simulink model "driveguard_simulation"  (R2023a)
settings: Solver=ode4  StartTime=0.0  StopTime=60  FixedStep=0.1  RelTol=1e-3
libraries: SignalEditorBlockLib x3, simulink x2
settings Model: Creator=Pulkit  LastModifiedBy=Pulkit

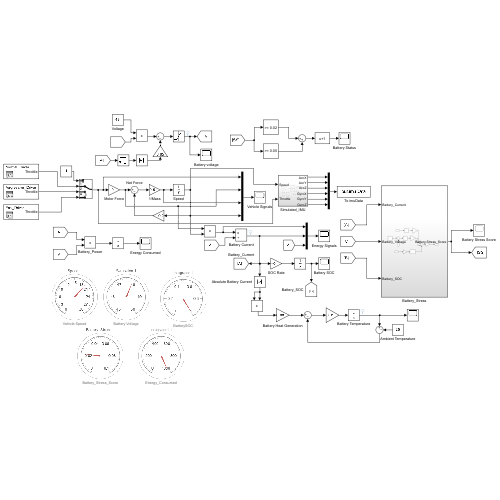
[thumbnail: Simulink's stored preview of the top-level diagram]
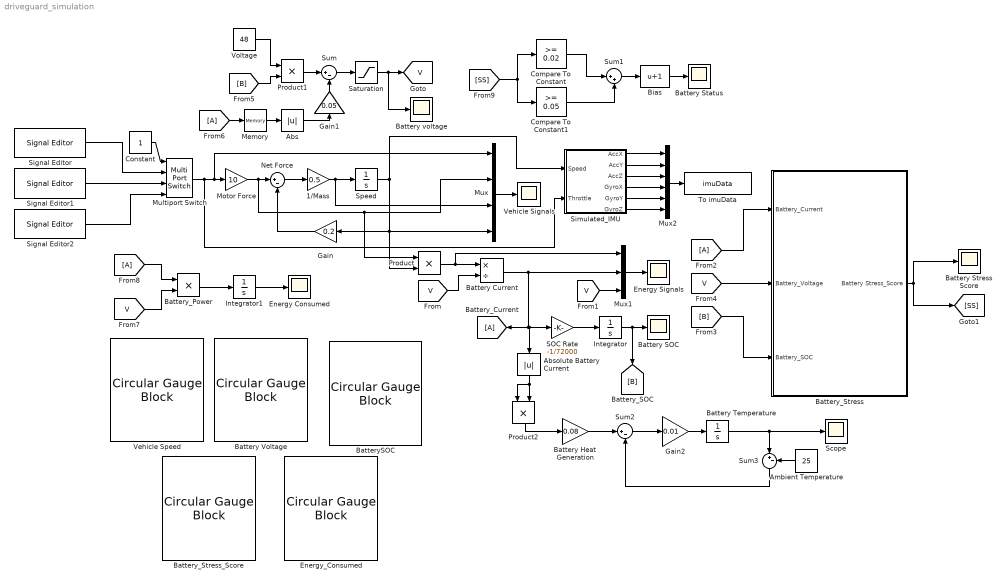
== system driveguard_simulation ==
  1/Mass : Gain  Gain=0.5
  Abs : Abs  SaturateOnIntegerOverflow=off
  Absolute Battery Current : Abs  SaturateOnIntegerOverflow=off
  Ambient Temperature : Constant  Value=25
  Battery Current : Product  Inputs=*/
  Battery Heat Generation : Gain  Gain=0.08
  Battery SOC : Scope
  Battery Status : Scope
  Battery Stress Score : Scope
  Battery Temperature : Integrator  InitialCondition=25
  Battery Voltage : CircularGaugeBlock  ScaleMin=45  ScaleMax=50  TickInterval=1
  Battery voltage : Scope
  BatterySOC : CircularGaugeBlock  ScaleMax=1  TickInterval=0.2
  Battery_Current : Goto
  Battery_Power : Product
  Battery_Stress : Subsystem
  Battery_Stress_Score : CircularGaugeBlock  ScaleMax=0.1  TickInterval=0.02
  Bias : Bias  Bias=1  SaturateOnIntegerOverflow=off
  Compare To Constant : simulink/Logic and Bit Operations/Compare To Constant  relop=>=  const=0.02  OutDataTypeStr=boolean
  Compare To Constant1 : simulink/Logic and Bit Operations/Compare To Constant  relop=>=  const=0.05  OutDataTypeStr=boolean
  Constant : Constant  SampleTime=-1
  Energy Consumed : Scope
  Energy Signals : Scope
  Energy_Consumed : CircularGaugeBlock  ScaleMax=1000  TickInterval=200
  From2 : From
  From6 : From
  From8 : From
  Gain : Gain  Gain=0.2
  Gain1 : Gain  Gain=0.05
  Gain2 : Gain  Gain=0.01
  Integrator : Integrator  InitialCondition=1
  Integrator1 : Integrator
  Memory : Memory
  Motor Force : Gain  Gain=10
  Multiport Switch : MultiPortSwitch  SaturateOnIntegerOverflow=off  InputSameDT=off
  Mux : Mux
  Mux1 : Mux  Inputs=3
  Mux2 : Mux  Inputs=6
  Net Force : Sum  Inputs=|+-
  Product : Product
  Product1 : Product
  Product2 : Product
  SOC Rate : Gain  Gain=-1/72000
  Saturation : Saturate  UpperLimit=100  LowerLimit=1
  Scope : Scope
  Signal Editor : SignalEditorBlockLib/Signal Editor  FileName=driver_profiles.mat  ActiveScenario=Normal_Driver  ActiveSignal=Throttle  IsBus=off  OutputBusObjectStr=Bus: BusObject  SampleTime=0  Interpolate=off  ZeroCross=off  OutputAfterFinalValue=Setting to zero  Unit=inherit  PreserveSignalName=on  ApplySigPropsToAllScenarios=on
  Signal Editor1 : SignalEditorBlockLib/Signal Editor  FileName=driver_profiles.mat  ActiveScenario=Aggressive_Driver  ActiveSignal=Throttle  IsBus=off  OutputBusObjectStr=Bus: BusObject  SampleTime=0  Interpolate=off  ZeroCross=off  OutputAfterFinalValue=Setting to zero  Unit=inherit  PreserveSignalName=on  ApplySigPropsToAllScenarios=on
  Signal Editor2 : SignalEditorBlockLib/Signal Editor  FileName=driver_profiles.mat  ActiveScenario=Eco_Driver  ActiveSignal=Throttle  IsBus=off  OutputBusObjectStr=Bus: BusObject  SampleTime=0  Interpolate=off  ZeroCross=off  OutputAfterFinalValue=Setting to zero  Unit=inherit  PreserveSignalName=on  ApplySigPropsToAllScenarios=on
  Simulated_IMU : Subsystem
  Speed : Integrator
  Sum : Sum  Inputs=|+-
  Sum1 : Sum  Inputs=|++
  Sum2 : Sum  Inputs=|+-
  Sum3 : Sum  Inputs=|+-
  To imuData : ToWorkspace  VariableName=imuData  SampleTime=-1
  Vehicle Signals : Scope
  Vehicle Speed : CircularGaugeBlock  ScaleMax=30  TickInterval=3
  Voltage : Constant  Value=48
  tag scope: V=global
  wires:
  1/Mass/1 -> Mux/3, Speed/1
  Speed/1 -> Gain/1, Product/2, Mux/4, Simulated_IMU/1(Speed)
  Motor Force/1 -> Product/1, Mux/2, Net Force/1
  Net Force/1 -> 1/Mass/1
  Gain/1 -> Net Force/2
  Mux/1 -> Vehicle Signals/1
  Product/1 -> Battery Current/1, Mux1/1
  Battery Current/1 -> SOC Rate/1, Absolute Battery Current/1, Battery_Current/1, Mux1/2
  Mux1/1 -> Energy Signals/1
  SOC Rate/1 -> Integrator/1
  Integrator/1 -> [B], Battery SOC/1
  [V] -> Battery Current/2
  [V] -> Mux1/3
  Signal Editor/1 -> Multiport Switch/2
  Signal Editor1/1 -> Multiport Switch/3
  Signal Editor2/1 -> Multiport Switch/4
  Multiport Switch/1 -> Simulated_IMU/2(Throttle), Mux/1, Motor Force/1
  Constant/1 -> Multiport Switch/1
  From2/1 -> Battery_Stress/1(Battery_Current)
  [V] -> Battery_Stress/2(Battery_Voltage)
  [B] -> Battery_Stress/3(Battery_SOC)
  Battery_Stress/1(Battery Stress_Score) -> Battery Stress Score/1, [SS]
  [B] -> Product1/2
  Abs/1 -> Gain1/1
  Product1/1 -> Sum/1
  Gain1/1 -> Sum/2
  From6/1 -> Memory/1
  Memory/1 -> Abs/1
  Voltage/1 -> Product1/1
  Sum/1 -> Saturation/1
  Saturation/1 -> Battery voltage/1, [V]
  From8/1 -> Battery_Power/1
  [V] -> Battery_Power/2
  Battery_Power/1 -> Integrator1/1
  Integrator1/1 -> Energy Consumed/1
  [SS] -> Compare To Constant1/1, Compare To Constant/1
  Compare To Constant/1 -> Sum1/1
  Compare To Constant1/1 -> Sum1/2
  Sum1/1 -> Bias/1
  Bias/1 -> Battery Status/1
  Absolute Battery Current/1 -> Product2/1, Product2/2
  Product2/1 -> Battery Heat Generation/1
  Battery Heat Generation/1 -> Sum2/1
  Sum2/1 -> Gain2/1
  Gain2/1 -> Battery Temperature/1
  Battery Temperature/1 -> Scope/1, Sum3/1
  Ambient Temperature/1 -> Sum3/2
  Sum3/1 -> Sum2/2
  Simulated_IMU/1(AccX) -> Mux2/1
  Simulated_IMU/2(AccY) -> Mux2/2
  Simulated_IMU/3(AccZ) -> Mux2/3
  Simulated_IMU/4(GyroX) -> Mux2/4
  Simulated_IMU/5(GyroY) -> Mux2/5
  Simulated_IMU/6(GyroZ) -> Mux2/6
  Mux2/1 -> To imuData/1

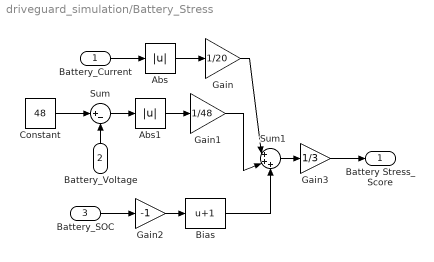
== system driveguard_simulation/Battery_Stress ==
  Battery_Current : Inport
  Battery_Voltage : Inport  Port=2
  Battery_SOC : Inport  Port=3
  Abs : Abs  SaturateOnIntegerOverflow=off
  Abs1 : Abs  SaturateOnIntegerOverflow=off
  Bias : Bias  Bias=1  SaturateOnIntegerOverflow=off
  Constant : Constant  Value=48
  Gain : Gain  Gain=1/20
  Gain1 : Gain  Gain=1/48
  Gain2 : Gain  Gain=-1
  Gain3 : Gain  Gain=1/3
  Sum : Sum  Inputs=|+-
  Sum1 : Sum  Inputs=|+++
  Battery Stress_Score : Outport
  wires:
  Battery_Current/1 -> Abs/1
  Abs/1 -> Gain/1
  Battery_Voltage/1 -> Sum/2
  Constant/1 -> Sum/1
  Battery_SOC/1 -> Gain2/1
  Gain2/1 -> Bias/1
  Gain/1 -> Sum1/1
  Gain1/1 -> Sum1/2
  Bias/1 -> Sum1/3
  Sum1/1 -> Gain3/1
  Gain3/1 -> Battery Stress_Score/1
  Sum/1 -> Abs1/1
  Abs1/1 -> Gain1/1

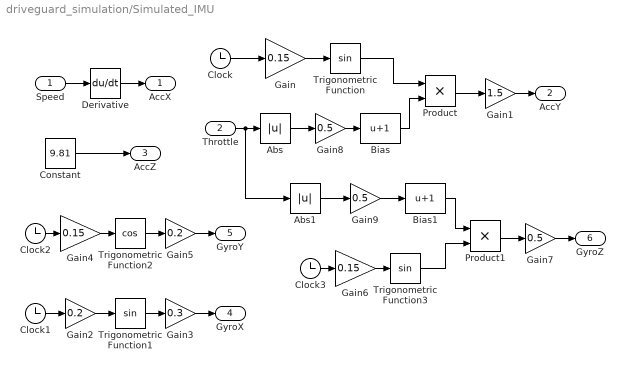
== system driveguard_simulation/Simulated_IMU ==
  Speed : Inport
  Throttle : Inport  Port=2
  Abs : Abs  SaturateOnIntegerOverflow=off
  Abs1 : Abs  SaturateOnIntegerOverflow=off
  Bias : Bias  Bias=1  SaturateOnIntegerOverflow=off
  Bias1 : Bias  Bias=1  SaturateOnIntegerOverflow=off
  Clock{,1..3} (4 alike) : Clock
  Constant : Constant  Value=9.81
  Derivative : Derivative
  Gain : Gain  Gain=0.15
  Gain1 : Gain  Gain=1.5
  Gain2 : Gain  Gain=0.2
  Gain3 : Gain  Gain=0.3
  Gain4 : Gain  Gain=0.15
  Gain5 : Gain  Gain=0.2
  Gain6 : Gain  Gain=0.15
  Gain7 : Gain  Gain=0.5
  Gain8 : Gain  Gain=0.5
  Gain9 : Gain  Gain=0.5
  Product : Product
  Product1 : Product
  Trigonometric Function : Trigonometry
  Trigonometric Function1 : Trigonometry
  Trigonometric Function2 : Trigonometry  Operator=cos
  Trigonometric Function3 : Trigonometry
  AccX : Outport
  AccY : Outport  Port=2
  AccZ : Outport  Port=3
  GyroX : Outport  Port=4
  GyroY : Outport  Port=5
  GyroZ : Outport  Port=6
  wires:
  Speed/1 -> Derivative/1
  Derivative/1 -> AccX/1
  Clock/1 -> Gain/1
  Gain/1 -> Trigonometric Function/1
  Gain1/1 -> AccY/1
  Constant/1 -> AccZ/1
  Clock1/1 -> Gain2/1
  Gain2/1 -> Trigonometric Function1/1
  Trigonometric Function1/1 -> Gain3/1
  Gain3/1 -> GyroX/1
  Clock2/1 -> Gain4/1
  Gain4/1 -> Trigonometric Function2/1
  Gain5/1 -> GyroY/1
  Trigonometric Function2/1 -> Gain5/1
  Gain7/1 -> GyroZ/1
  Gain6/1 -> Trigonometric Function3/1
  Clock3/1 -> Gain6/1
  Throttle/1 -> Abs1/1, Abs/1
  Trigonometric Function/1 -> Product/1
  Product/1 -> Gain1/1
  Abs/1 -> Gain8/1
  Gain8/1 -> Bias/1
  Bias/1 -> Product/2
  Abs1/1 -> Gain9/1
  Gain9/1 -> Bias1/1
  Trigonometric Function3/1 -> Product1/2
  Bias1/1 -> Product1/1
  Product1/1 -> Gain7/1
